simulink model "PID_Controller"  (R2024b)
settings: Solver=VariableStepAuto  StartTime=0.0  StopTime=10  RelTol=1e-3
settings Model: Creator=lpdtd  LastModifiedBy=lpdtd

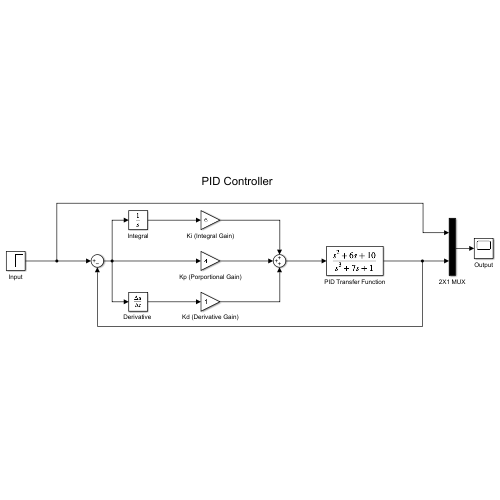
[thumbnail: Simulink's stored preview of the top-level diagram]
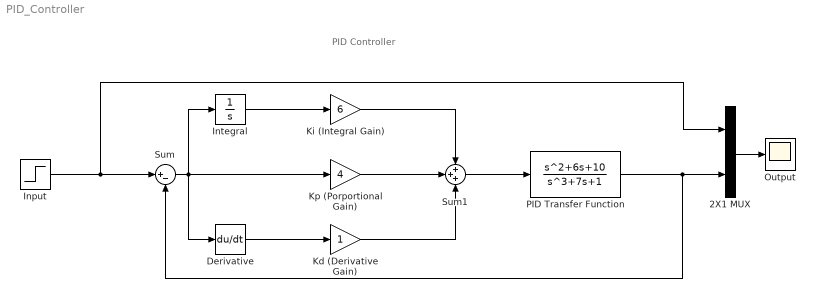
== system PID_Controller ==
  note: PID Controller
  2X1 MUX : Mux  Inputs=2
  "Derivative " : Derivative
  Input : Step  SampleTime=0
  Integral : Integrator
  Kd (Derivative Gain) : Gain
  Ki (Integral Gain) : Gain  Gain=6
  Kp (Porportional Gain) : Gain  Gain=4
  Output : Scope
  PID Transfer Function : TransferFcn  Numerator=[1,6,10]  Denominator=[1,0,7,1]
  Sum : Sum  Inputs=|+-
  Sum1 : Sum  Inputs=+++
  wires:
  2X1 MUX/1 -> Output/1
  Sum/1 -> "Derivative "/1, Integral/1, Kp (Porportional Gain)/1
  Input/1 -> 2X1 MUX/1, Sum/1
  PID Transfer Function/1 -> Sum/2, 2X1 MUX/2
  Kp (Porportional Gain)/1 -> Sum1/2
  Integral/1 -> Ki (Integral Gain)/1
  Ki (Integral Gain)/1 -> Sum1/1
  "Derivative "/1 -> Kd (Derivative Gain)/1
  Kd (Derivative Gain)/1 -> Sum1/3
  Sum1/1 -> PID Transfer Function/1
